simulink model "exp8"  (R2025b)
settings: Solver=VariableStepAuto  StartTime=0.0  StopTime=10.0  RelTol=1e-3
libraries: simulink_extras x5
settings Model: Creator=SUBHASH  LastModifiedBy=SUBHASH

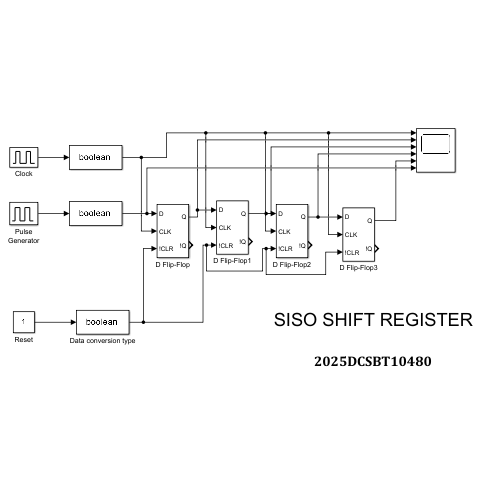
[thumbnail: Simulink's stored preview of the top-level diagram]
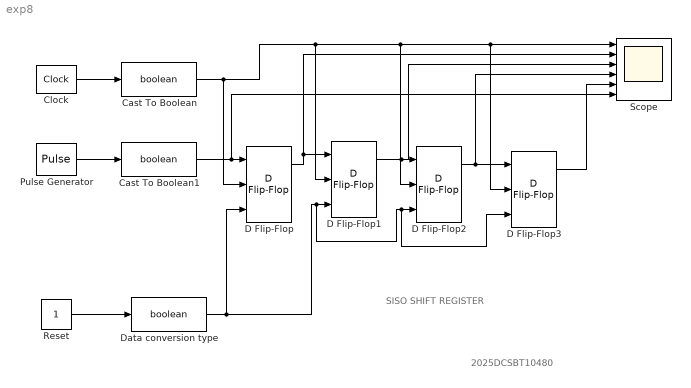
== system exp8 ==
  note: 2025DCSBT10480
  note: SISO SHIFT REGISTER
  Cast To Boolean : DataTypeConversion  OutDataTypeStr=boolean  SaturateOnIntegerOverflow=off  RndMeth=Floor
  Cast To Boolean1 : DataTypeConversion  OutDataTypeStr=boolean  SaturateOnIntegerOverflow=off  RndMeth=Floor
  Clock : simulink_extras/Flip Flops/Clock  period=2
  D Flip-Flop{,1..3} (4 alike) : simulink_extras/Flip Flops/D Flip-Flop
  Data conversion type : DataTypeConversion  OutDataTypeStr=boolean  SaturateOnIntegerOverflow=off  RndMeth=Floor
  Pulse Generator : DiscretePulseGenerator  PulseType=Time based  Period=10  PulseWidth=30
  Reset : Constant
  Scope : Scope  NumInputPorts=6
      settings: ActiveDisplayYMinimum=-0.12499999999999997  ActiveDisplayYMaximum=1.125
  wires:
  Clock/1 -> Cast To Boolean/1
  Cast To Boolean/1 -> D Flip-Flop/2, D Flip-Flop1/2, D Flip-Flop2/2, D Flip-Flop3/2, Scope/1
  Reset/1 -> Data conversion type/1
  Data conversion type/1 -> D Flip-Flop3/3, D Flip-Flop2/3, D Flip-Flop1/3, D Flip-Flop/3
  Pulse Generator/1 -> Cast To Boolean1/1
  Cast To Boolean1/1 -> Scope/6, D Flip-Flop/1
  D Flip-Flop/1 -> Scope/2, D Flip-Flop1/1
  D Flip-Flop1/1 -> Scope/3, D Flip-Flop2/1
  D Flip-Flop2/1 -> Scope/4, D Flip-Flop3/1
  D Flip-Flop3/1 -> Scope/5
